simulink model "simulation_regelkreis"  (Simulink 7.0)
settings: Solver=ode45  StartTime=0.0  StopTime=25.0  RelTol=1e-3
libraries: dspsrcs4 x1
settings Model: Creator=Matze  LastModifiedBy=Matze

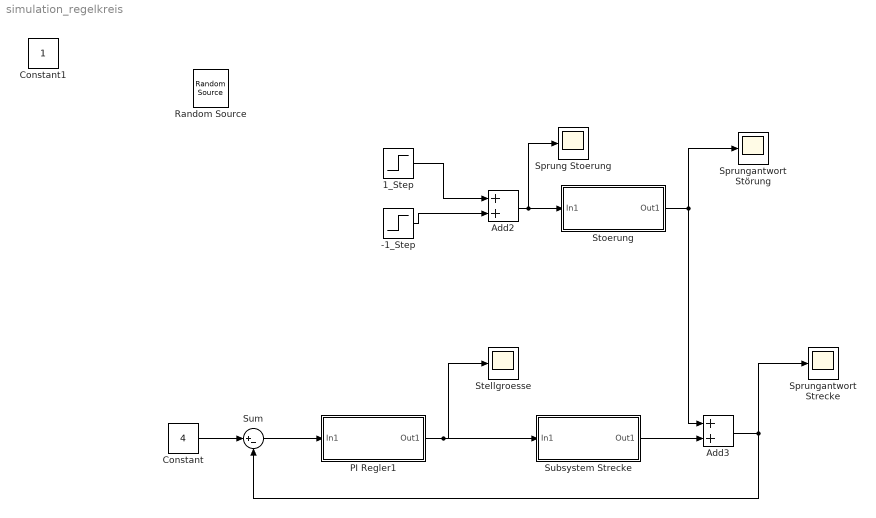
== system simulation_regelkreis ==
  -1_Step : Step  Time=9  After=-0.35  SampleTime=0
  1_Step : Step  Time=4.5  After=0.35  SampleTime=0
  Add2 : Sum  OutDataType=sfix(16)  OutScaling=2^-10
  Add3 : Sum  OutDataType=sfix(16)  OutScaling=2^-10
  Constant : Constant  Value=4  OutDataType=sfix(16)  OutScaling=2^0
  PI Regler1 : Subsystem
  Sprung Stoerung : Scope
      settings: TimeRange=10  YMin=0  SaveName=ScopeData2
  Sprungantwort Strecke : Scope
      settings: TimeRange=10  YMin=0  SaveName=ScopeData4
  Sprungantwort Störung : Scope
      settings: TimeRange=10  YMin=0
  Stellgroesse : Scope
      settings: TimeRange=10  YMin=0  SaveName=ScopeData5
  Stoerung : Subsystem
  Subsystem Strecke : Subsystem
  Sum : Sum  Inputs=|+-  OutDataType=sfix(16)  OutScaling=2^0
  Constant1 : Constant  IOType=siggen  OutDataType=sfix(16)  OutScaling=2^0
  Random Source : dspsrcs4/Random Source  IOType=siggen  SrcType=Uniform  NormMethod=Ziggurat  CltLength=12  MinVal=0  MaxVal=1  MeanVal=0  VarVal=1  RepMode=Not repeatable  rawSeed=1  IsInherit=off  SampMode=Discrete  SampTime=1  SampFrame=1  DataType=Double  OutComplex=Real
  wires:
  Constant/1 -> Sum/1
  1_Step/1 -> Add2/1
  -1_Step/1 -> Add2/2
  Add2/1 -> Stoerung/1(In1), Sprung Stoerung/1
  Stoerung/1(Out1) -> Add3/1, Sprungantwort Störung/1
  Subsystem Strecke/1(Out1) -> Add3/2
  Add3/1 -> Sprungantwort Strecke/1, Sum/2
  Sum/1 -> PI Regler1/1(In1)
  PI Regler1/1(Out1) -> Stellgroesse/1, Subsystem Strecke/1(In1)

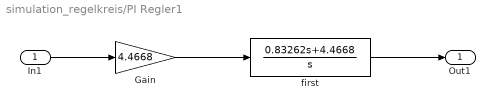
== system simulation_regelkreis/PI Regler1 ==
  In1 : Inport  OutDataType=sfix(16)  OutScaling=2^0
  Gain : Gain  Gain=4.4668  ParameterDataType=sfix(16)  ParameterScaling=2^0  OutDataType=sfix(16)  OutScaling=2^0
  first : TransferFcn  Numerator=[0.83262 4.4668]  Denominator=[1 0]
  Out1 : Outport  OutDataType=sfix(16)  OutScaling=2^0
  wires:
  In1/1 -> Gain/1
  first/1 -> Out1/1
  Gain/1 -> first/1

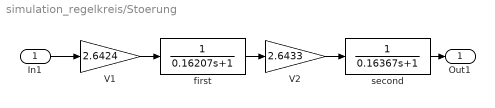
== system simulation_regelkreis/Stoerung ==
  In1 : Inport  OutDataType=sfix(16)  OutScaling=2^0
  V1 : Gain  Gain=2.6424  ParameterDataType=sfix(16)  ParameterScaling=2^0  OutDataType=sfix(16)  OutScaling=2^0
  V2 : Gain  Gain=2.6433  ParameterDataType=sfix(16)  ParameterScaling=2^0  OutDataType=sfix(16)  OutScaling=2^0
  first : TransferFcn  Denominator=[0.16207 1]
  second : TransferFcn  Denominator=[0.16367 1]
  Out1 : Outport  OutDataType=sfix(16)  OutScaling=2^0
  wires:
  In1/1 -> V1/1
  V1/1 -> first/1
  first/1 -> V2/1
  second/1 -> Out1/1
  V2/1 -> second/1

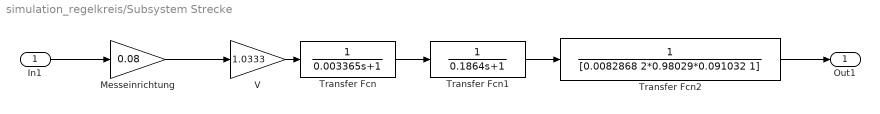
== system simulation_regelkreis/Subsystem Strecke ==
  In1 : Inport  OutDataType=sfix(16)  OutScaling=2^0
  Messeinrichtung : Gain  Gain=0.08  ParameterDataType=sfix(16)  ParameterScaling=2^0  OutDataType=sfix(16)  OutScaling=2^0
  Transfer Fcn : TransferFcn  Denominator=[0.003365 1]
  Transfer Fcn1 : TransferFcn  Denominator=[0.1864 1]
  Transfer Fcn2 : TransferFcn  Denominator=[0.0082868 2*0.98029*0.091032 1]
  V : Gain  Gain=1.0333  ParameterDataType=sfix(16)  ParameterScaling=2^0  OutDataType=sfix(16)  OutScaling=2^0
  Out1 : Outport  OutDataType=sfix(16)  OutScaling=2^0
  wires:
  In1/1 -> Messeinrichtung/1
  V/1 -> Transfer Fcn/1
  Transfer Fcn/1 -> Transfer Fcn1/1
  Transfer Fcn1/1 -> Transfer Fcn2/1
  Transfer Fcn2/1 -> Out1/1
  Messeinrichtung/1 -> V/1
